simulink model "pendulum_sim"  (R2024a)
settings: Solver=VariableStepAuto  StartTime=0.0  StopTime=t_sim  RelTol=1e-3
values from neighbouring files (symbols this model uses):
  beta = 0.6    [pendulum.m]
  J = m*l^2    (= 0.64)    [pendulum.m]
  K = 9.8*m*l    (= 7.84)    [pendulum.m]
settings Model: Creator=lorenzo  LastModifiedBy=lorenzo

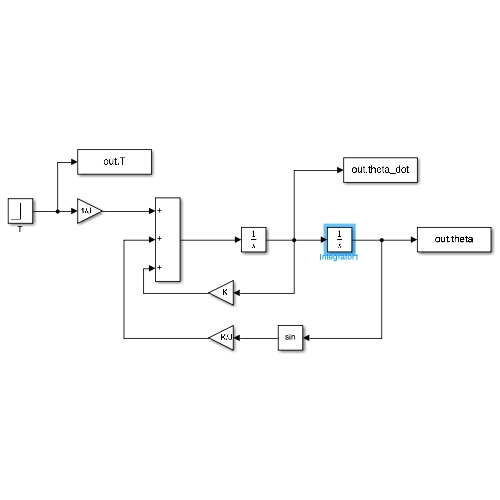
[thumbnail: Simulink's stored preview of the top-level diagram]
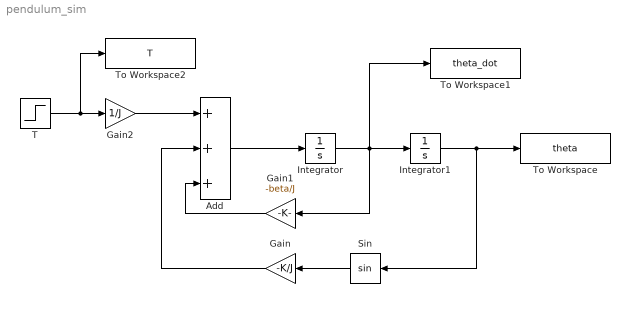
== system pendulum_sim ==
  Add : Sum  Inputs=+++
  Gain : Gain  Gain=-K/J
  Gain1 : Gain  Gain=-beta/J
  Gain2 : Gain  Gain=1/J
  Integrator : Integrator
  Integrator1 : Integrator  InitialCondition=[pi/4]
  Sin : Trigonometry
  T : Step  Time=0  After=0  SampleTime=0
  To Workspace : ToWorkspace  VariableName=theta  SaveFormat=Timeseries  SampleTime=-1
  To Workspace1 : ToWorkspace  VariableName=theta_dot  SaveFormat=Timeseries  SampleTime=-1
  To Workspace2 : ToWorkspace  VariableName=T  SaveFormat=Timeseries  SampleTime=-1
  wires:
  Integrator1/1 -> Sin/1, To Workspace/1
  Sin/1 -> Gain/1
  Add/1 -> Integrator/1
  Gain2/1 -> Add/1
  Gain1/1 -> Add/3
  Gain/1 -> Add/2
  T/1 -> Gain2/1, To Workspace2/1
  Integrator/1 -> To Workspace1/1, Gain1/1, Integrator1/1
